simulink model "RudderActuatorChannel_control_lin"  (R2015a)
settings: Solver=ode4  SolverMode=SingleTasking  StartTime=0.0  StopTime=2.999  FixedStep=sampleTime  MaxStep=1e-3  MinStep=1e-4
undefined symbols (not defined in the file or in its folder): Acv, Aleak1, Aleak2, Aleak3, Aleak4, Aleak5, Aleakext, Aleakint, Ap, Ap_seal, Ar_seal, As_ehsv, Be, Bkp_seal, Bp1, C, Cd, ControlTopology, DeltaQ_ehsv, EHSV_Step, ent_air, frictionstribeck_velocity, gamma_air, i_ehsv, Imax, Input, K2_ehsv, K3_ehsv, K_Supply1, Ka1, Kd, Ki, Ki_ehsv, Kp, Kr_ehsv, ksi_ehsv, Kst, Kst_Enable, Kw_ehsv, L0, Load_cmd, Lp_seal, Lr_seal, Max_Cmd, Min_Cmd, Mp1, ON_OFF_hyst, P10, Pcvac, Pcvi, Pcvr, Ps0, Pt0, Ql_ehsv, R, Rate_Limit, Return_Pressure, Rho, sampleTime, seal_compression ... (+20)
undefined symbols (not defined in the file): dpLVDT, Kd_N, ramLVDT, xvLVDT
libraries: simulink x1
(part 1 of 2)
settings Model: SimulationMode=accelerator  Creator=Charles  LastModifiedBy=Pedro H
settings SolverCC: InitialStep=1e-4
settings DataIOCC: LimitDataPoints=off  SaveFormat=StructureWithTime  DSMLogging=off  SaveTime=off
settings OptimizationCC: ExpressionDepthLimit=2147483647  InitFltsAndDblsToZero=on
settings DebuggingCC: SaveWithParameterizedLinksMsg=none  UnderspecifiedInitializationDetection=Classic  MergeDetectMultiDrivingBlocksExec=none  SolverPrmCheckMsg=warning  InheritedTsInSrcMsg=none  FcnCallInpInsideContextMsg=UseLocalSettings  StateNameClashWarn=warning
settings ModelReferenceCC: UpdateModelReferenceTargets=IfOutOfDate
settings GRTTargetCC: TargetFcnLib=ansi_tfl_tmw.mat  CombineOutputUpdateFcns=off  GRTInterface=on

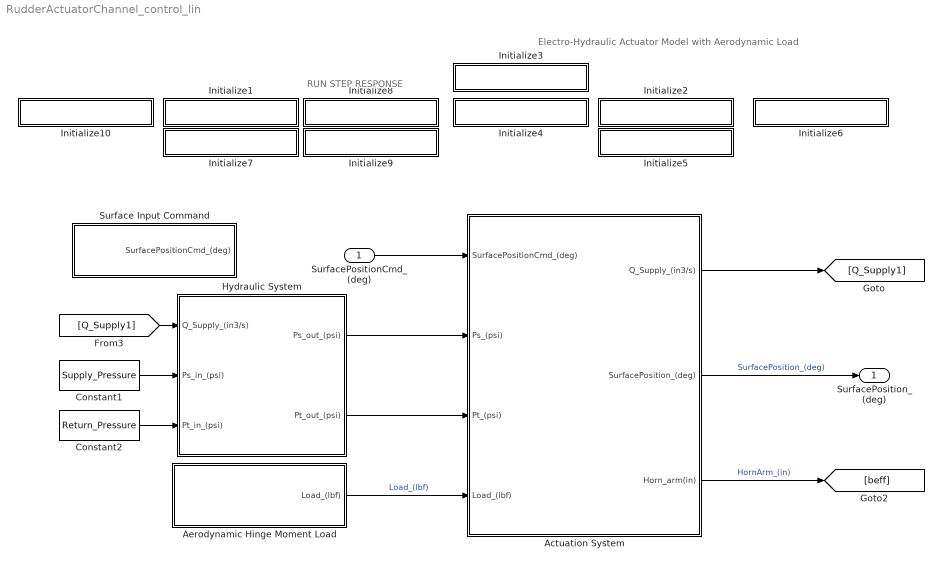
== system RudderActuatorChannel_control_lin ==
  note: RUN STEP RESPONSE
  note: Electro-Hydraulic Actuator Model with Aerodynamic Load
  SurfacePositionCmd_(deg) : Inport
  Actuation System : Subsystem
  Aerodynamic Hinge Moment Load : Subsystem
  Constant1 : Constant  Value=Supply_Pressure
  Constant2 : Constant  Value=Return_Pressure
  Hydraulic System : Subsystem
  Initialize1 : Subsystem
      settings: OpenFcn=|
      | run('StepInput_CLLoad.m'),
      | set_param(bdroot,'SimulationCommand','start')
      mask Display: disp('Closed Loop - Loaded')
  Initialize10 : Subsystem
      settings: OpenFcn=|
      | run('SineInput_CLLoad.m'),
      | set_param(bdroot,'SimulationCommand','start')
      mask Display: disp('Run Sine Input')
  Initialize2 : Subsystem
      settings: OpenFcn=|
      | FreqResp_type = 0;
      | run('FrequencyResponseTest.m'),
      | set_param(bdroot,'SimulationCommand','start')
      mask Display: disp('Frequency Response')
  Initialize3 : Subsystem
      settings: OpenFcn=run('Load_Parameters.m'),
      mask Display: disp('Model Initialization')
  Initialize4 : Subsystem
      settings: OpenFcn=run('plotMaster.m')
      mask Display: disp('Plot Results')
  Initialize5 : Subsystem
      settings: OpenFcn=|
      | FreqResp_type = 1;
      | run('FrequencyResponseTest.m'),
      | set_param(bdroot,'SimulationCommand','start')
      mask Display: disp('Run EHSV Frequency Response Test')
  Initialize6 : Subsystem
      settings: OpenFcn=run('DynamicStiffnessTest.m')
      mask Display: disp('Dynamic Stiffness Test')
  Initialize7 : Subsystem
      settings: OpenFcn=|
      | run('StepInput_CLNoLoad.m'),
      | set_param(bdroot,'SimulationCommand','start')
      mask Display: disp('Closed Loop - Unloaded')
  Initialize8 : Subsystem
      settings: OpenFcn=|
      | run('StepInput_OLEHSVLoad.m'),
      | set_param(bdroot,'SimulationCommand','start')
      mask Display: disp('Open Loop - Loaded')
  Initialize9 : Subsystem
      settings: OpenFcn=|
      | run('StepInput_OLEHSVNoLoad.m'),
      | set_param(bdroot,'SimulationCommand','start')
      mask Display: disp('Open Loop - Unloaded')
  Surface Input Command : Subsystem
  SurfacePosition_(deg) : Outport
  wires:
  Constant1/1 -> Hydraulic System/2(Ps_in_(psi))
  Constant2/1 -> Hydraulic System/3(Pt_in_(psi))
  Hydraulic System/1(Ps_out_(psi)) -> Actuation System/2(Ps_(psi))
  Hydraulic System/2(Pt_out_(psi)) -> Actuation System/3(Pt_(psi))
  Actuation System/1(Q_Supply_(in3/s)) -> [Q_Supply1]
  [Q_Supply1] -> Hydraulic System/1(Q_Supply_(in3/s))
  Actuation System/2(SurfacePosition_(deg)) -> SurfacePosition_(deg)/1  "SurfacePosition_(deg)"
  Actuation System/3(Horn_arm(in)) -> [beff]  "HornArm_(in)"
  Aerodynamic Hinge Moment Load/1(Load_(lbf)) -> Actuation System/4(Load_(lbf))  "Load_(lbf)"
  SurfacePositionCmd_(deg)/1 -> Actuation System/1(SurfacePositionCmd_(deg))

== system RudderActuatorChannel_control_lin/Actuation System ==
  SurfacePositionCmd_(deg) : Inport
  Ps_(psi) : Inport  Port=2
  Pt_(psi) : Inport  Port=3
  Load_(lbf) : Inport  Port=4
  Actuator : Subsystem
  Bus Creator : BusCreator  Inputs=2  OutDataTypeStr=Bus: ActSysHydPower  NonVirtualBus=on
  Electronics System : Subsystem
  Scope : Scope
      settings: SaveName=ScopeData6
  Surface Kinematics : Subsystem
  Q_Supply_(in3/s) : Outport
  SurfacePosition_(deg) : Outport  Port=2
  Horn_arm(in) : Outport  Port=3
  wires:
  [Sensors_FB] -> Electronics System/2(Sensors_FB)
  SurfacePositionCmd_(deg)/1 -> Electronics System/1(Theta_Cmd_(deg))
  Ps_(psi)/1 -> Bus Creator/1  "Ps"
  Pt_(psi)/1 -> Bus Creator/2  "Pt"
  Bus Creator/1 -> Actuator/3(Hyd_Power)
  Actuator/2(Q_Supply) -> Q_Supply_(in3/s)/1
  Actuator/1(Xp_real_(in)) -> Surface Kinematics/1(Xp_(in))  "Xp"
  Load_(lbf)/1 -> [Load]
  Surface Kinematics/1(ThetaPos_(deg)) -> SurfacePosition_(deg)/1
  Actuator/3(Sensors) -> [Sensors_FB]
  Surface Kinematics/2(Effective_arm_(in)) -> Horn_arm(in)/1
  [Load] -> Scope/1, Actuator/2(Load)
  Electronics System/1(Current_Cmd_(mA)) -> Actuator/1(Current_Cmd)

== system RudderActuatorChannel_control_lin/Aerodynamic Hinge Moment Load ==
  Constant2 : Constant  Value=Load_cmd
  Load_(lbf) : Outport
  wires:
  Constant2/1 -> Load_(lbf)/1

== system RudderActuatorChannel_control_lin/Hydraulic System ==
  Q_Supply_(in3/s) : Inport
  Ps_in_(psi) : Inport  Port=2
  Pt_in_(psi) : Inport  Port=3
  Aircraft Hydraulic Losses : Gain  Gain=K_Supply1
  Bus Selector : BusSelector  OutputSignals=Qs
  Fluid Inertia : TransferFcn  Denominator=[0.01 1]
  Sum1 : Sum  Inputs=|+-
  cis to gpm : Gain  Gain=0.25974
  Ps_out_(psi) : Outport
  Pt_out_(psi) : Outport  Port=2
  wires:
  Sum1/1 -> Ps_out_(psi)/1  "Ps"
  Aircraft Hydraulic Losses/1 -> Fluid Inertia/1
  Fluid Inertia/1 -> Sum1/2
  Pt_in_(psi)/1 -> Pt_out_(psi)/1  "Pt"
  Ps_in_(psi)/1 -> Sum1/1  "Ps"
  Q_Supply_(in3/s)/1 -> Bus Selector/1
  cis to gpm/1 -> Aircraft Hydraulic Losses/1
  Bus Selector/1 -> cis to gpm/1  "<Qs>"

== system RudderActuatorChannel_control_lin/Initialize1 ==

== system RudderActuatorChannel_control_lin/Initialize10 ==

== system RudderActuatorChannel_control_lin/Initialize2 ==

== system RudderActuatorChannel_control_lin/Initialize3 ==

== system RudderActuatorChannel_control_lin/Initialize4 ==

== system RudderActuatorChannel_control_lin/Initialize5 ==

== system RudderActuatorChannel_control_lin/Initialize6 ==

== system RudderActuatorChannel_control_lin/Initialize7 ==

== system RudderActuatorChannel_control_lin/Initialize8 ==

== system RudderActuatorChannel_control_lin/Initialize9 ==

== system RudderActuatorChannel_control_lin/Surface Input Command ==
  Step1 : Step  Time=Input.Step.Time  Before=Input.Step.InitialValue  After=Input.Step.FinalValue  SampleTime=0
  SurfacePositionCmd_(deg) : Outport
  wires:
  Step1/1 -> SurfacePositionCmd_(deg)/1

== system RudderActuatorChannel_control_lin/Actuation System/Actuator ==
  Current_Cmd : Inport
  Load : Inport  Port=2
  Hyd_Power : Inport  Port=3
  Cylinder Dynamics : Subsystem
  Sensors Dynamics : Subsystem
  Valves Dynamics : Subsystem
  Xp_real_(in) : Outport
  Q_Supply : Outport  Port=2
  Sensors : Outport  Port=3
  wires:
  Cylinder Dynamics/2(Xp) -> Xp_real_(in)/1, [Xp]
  Load/1 -> Cylinder Dynamics/2(Load)
  Valves Dynamics/2(Q_Supply) -> Q_Supply/1
  Valves Dynamics/1(Q_Act) -> Cylinder Dynamics/1(Q_Act)
  Current_Cmd/1 -> Valves Dynamics/2(Currrent)
  Hyd_Power/1 -> Valves Dynamics/3(Hyd_Pwr)
  Cylinder Dynamics/1(P_Act) -> Valves Dynamics/1(P_Act)
  Cylinder Dynamics/3(Qacv) -> Valves Dynamics/4(Qacv)
  Valves Dynamics/3(Pt) -> Cylinder Dynamics/3(Pt)
  Valves Dynamics/4(Xv_(in)) -> [Xv]
  Cylinder Dynamics/4(dP) -> [dP]
  [Xp] -> Sensors Dynamics/1(Xp)
  [dP] -> Sensors Dynamics/2(dP)
  [Xv] -> Sensors Dynamics/3(Xv)
  Sensors Dynamics/1(Sensors) -> Sensors/1

== system RudderActuatorChannel_control_lin/Actuation System/Electronics System ==
  Theta_Cmd_(deg) : Inport
  Sensors_FB : Inport  Port=2
  Digital Controller : Subsystem
  Hardware_in : Subsystem
  Hardware_out : Subsystem
  Current_Cmd_(mA) : Outport
  wires:
  Theta_Cmd_(deg)/1 -> Hardware_in/1(Theta_Cmd_in)
  Digital Controller/1(EHSV_Cmd) -> Hardware_out/1(EHSV_Cmd_in)
  Hardware_in/1(Theta_Cmd_out) -> Digital Controller/1(Cmd_D)
  Hardware_in/2(Sensors_FB_out) -> Digital Controller/2(Sensors_FB)
  Sensors_FB/1 -> Hardware_in/2(Sensors_FB_in)
  Hardware_out/1(EHSV_Cmd_out) -> Current_Cmd_(mA)/1

== system RudderActuatorChannel_control_lin/Actuation System/Surface Kinematics ==
  Xp_(in) : Inport
  Rad2Deg : Gain  Gain=180/pi  SaturateOnIntegerOverflow=on  OutDataTypeStr=Inherit: Same as input  ParamDataTypeStr=Inherit: Same as input
  Real Kinematics : Subsystem
  ThetaPos_(deg) : Outport
  Effective_arm_(in) : Outport  Port=2
  wires:
  Xp_(in)/1 -> Real Kinematics/1(Xp)
  Real Kinematics/1(Theta) -> Rad2Deg/1
  Rad2Deg/1 -> ThetaPos_(deg)/1
  Real Kinematics/2(Reff) -> Effective_arm_(in)/1

== system RudderActuatorChannel_control_lin/Actuation System/Actuator/Cylinder Dynamics ==
  Q_Act : Inport
  Load : Inport  Port=2
  Pt : Inport  Port=3
  Bus Creator1 : BusCreator  Inputs=2  OutDataTypeStr=Bus: CYLQacv  NonVirtualBus=on
  Bus Creator3 : BusCreator  Inputs=2  OutDataTypeStr=Bus: CYLPAct  NonVirtualBus=on
  Bus Selector : BusSelector  OutputSignals=Q1,Q2
  Fluid Dynamics : Subsystem
  Piston Dynamics : Subsystem
  Scope : Scope  NumInputPorts=5
      settings: YMin=-5~-5~-5~-5~-5  YMax=5~5~5~5~5  SaveName=ScopeData8
  P_Act : Outport
  Xp : Outport  Port=2
  Qacv : Outport  Port=3
  dP : Outport  Port=4
  wires:
  Bus Creator3/1 -> P_Act/1
  Q_Act/1 -> Bus Selector/1
  Bus Selector/2 -> Fluid Dynamics/4(Q2)  "<Q2>"
  Piston Dynamics/1(Xp) -> [Xp], Xp/1
  Piston Dynamics/2(Xpdot) -> [Xpdot]  "Xpdot"
  [Xp] -> Scope/3, Fluid Dynamics/1(xp)
  [Xpdot] -> Scope/4, Fluid Dynamics/2(xpdot)
  Load/1 -> Piston Dynamics/3(FL)
  Bus Selector/1 -> Fluid Dynamics/3(Q1)  "<Q1>"
  Fluid Dynamics/2(P2) -> Scope/2, Piston Dynamics/2(Pr), Bus Creator3/2  "P2"
  Fluid Dynamics/1(P1) -> Scope/1, Piston Dynamics/1(Pe), Bus Creator3/1  "P1"
  Pt/1 -> Fluid Dynamics/5(Pt)
  Fluid Dynamics/3(Qacv1) -> Bus Creator1/1  "Qacv1"
  Fluid Dynamics/4(Qacv2) -> Bus Creator1/2  "Qacv2"
  Bus Creator1/1 -> Qacv/1
  Fluid Dynamics/5(dP) -> Scope/5, dP/1

== system RudderActuatorChannel_control_lin/Actuation System/Actuator/Sensors Dynamics ==
  Xp : Inport
  dP : Inport  Port=2
  Xv : Inport  Port=3
  Bus Creator : BusCreator  Inputs=3  OutDataTypeStr=Bus: SensorDyn  NonVirtualBus=on
  "Xp LVDT " : Subsystem
  "Xv LVDT " : Subsystem
  "dP LVDT " : Subsystem
  Sensors : Outport
  wires:
  dP/1 -> "dP LVDT "/1(dP_real)
  Xp/1 -> "Xp LVDT "/1(Xp_real)
  Xv/1 -> "Xv LVDT "/1(Xv_real)
  "Xv LVDT "/1(Xv_LVDT) -> Bus Creator/3  "Xv_mesured_(in)"
  "dP LVDT "/1(dP_LVDT) -> Bus Creator/2  "dP_mesured_(psi)"
  "Xp LVDT "/1(Xp_LVDT) -> Bus Creator/1  "Xp_mesured_(in)"
  Bus Creator/1 -> Sensors/1

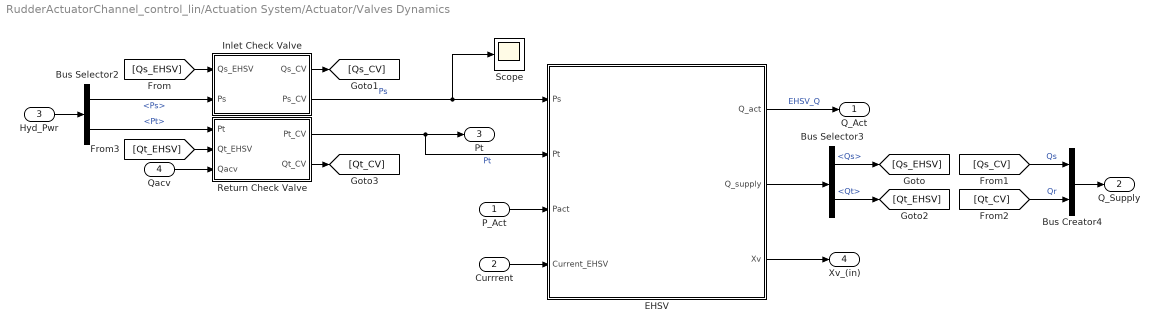
== system RudderActuatorChannel_control_lin/Actuation System/Actuator/Valves Dynamics ==
  P_Act : Inport
  Currrent : Inport  Port=2
  Hyd_Pwr : Inport  Port=3
  Qacv : Inport  Port=4
  Bus Creator4 : BusCreator  Inputs=2  OutDataTypeStr=Bus: VALVEOutQSup  NonVirtualBus=on
  Bus Selector2 : BusSelector  OutputSignals=Ps,Pt
  Bus Selector3 : BusSelector  OutputSignals=Qs,Qt
  EHSV : Subsystem
  Inlet Check Valve : Subsystem
  Return Check Valve : Subsystem
  Scope : Scope
      settings: SaveName=ScopeData5
  Q_Act : Outport
  Q_Supply : Outport  Port=2
  Pt : Outport  Port=3
  Xv_(in) : Outport  Port=4
  wires:
  Hyd_Pwr/1 -> Bus Selector2/1
  EHSV/1(Q_act) -> Q_Act/1  "EHSV_Q"
  Bus Selector2/1 -> Inlet Check Valve/2(Ps)  "<Ps>"
  Bus Selector3/1 -> [Qs_EHSV]  "<Qs>"
  [Qs_EHSV] -> Inlet Check Valve/1(Qs_EHSV)
  Inlet Check Valve/1(Qs_CV) -> [Qs_CV]
  [Qs_CV] -> Bus Creator4/1  "Qs"
  Bus Creator4/1 -> Q_Supply/1
  Bus Selector2/2 -> Return Check Valve/1(Pt)  "<Pt>"
  Bus Selector3/2 -> [Qt_EHSV]  "<Qt>"
  [Qt_CV] -> Bus Creator4/2  "Qr"
  [Qt_EHSV] -> Return Check Valve/2(Qt_EHSV)
  Return Check Valve/2(Qt_CV) -> [Qt_CV]
  Qacv/1 -> Return Check Valve/3(Qacv)
  Currrent/1 -> EHSV/4(Current_EHSV)
  P_Act/1 -> EHSV/3(Pact)
  Inlet Check Valve/2(Ps_CV) -> Scope/1, EHSV/1(Ps)  "Ps"
  Return Check Valve/1(Pt_CV) -> EHSV/2(Pt), Pt/1  "Pt"
  EHSV/2(Q_supply) -> Bus Selector3/1
  EHSV/3(Xv) -> Xv_(in)/1

== system RudderActuatorChannel_control_lin/Actuation System/Electronics System/Digital Controller ==
  Cmd_D : Inport
  Sensors_FB : Inport  Port=2
  Bus Selector : BusSelector  OutputSignals=Xp_FB
  Command Limits : Saturate  UpperLimit=Max_Cmd  LowerLimit=Min_Cmd
  Constant : Constant  Value=ControlTopology
  Constant1 : Constant
  Constant2 : Constant  Value=2
  Deg2Rad : Gain  Gain=pi/180  SampleTime=T_ES  SaturateOnIntegerOverflow=on  OutDataTypeStr=Inherit: Same as input  ParamDataTypeStr=Inherit: Same as input
  Kinematics : Subsystem
  LQR : Subsystem  mask{K=[14.6507 0.0003   22.9112 ]}
      mask prompts: K "State Control gain (K)"
  Manual Switch : ManualSwitch  CurrentSetting=0
  Multiport Switch : MultiPortSwitch  Inputs=5
  On-Off Controller : Relay  OnSwitchValue=ON_OFF_hyst  OffSwitchValue=-ON_OFF_hyst  OnOutputValue=10  OffOutputValue=-10
  PID controller : Subsystem  mask{Kp=Kp, Ki=Ki, Kd=Kd, Ts=T_ES, kd_N=Kd_N, umax=10}
      mask prompts: Ts "Sampling Time"; kd_N "Kd Filter coefficient"; umax "Max command"
  Rate Limit : Subsystem
  Saturation +/- 10mA : Saturate  UpperLimit=Imax  LowerLimit=-Imax  SampleTime=T_ES
  Scope : Scope
  Scope1 : Scope
      settings: SaveName=ScopeData2
  Sgn Convention : Gain  SampleTime=T_ES  SaturateOnIntegerOverflow=on  OutDataTypeStr=Inherit: Same as input  ParamDataTypeStr=Inherit: Same as input
  Step : Step  Time=EHSV_Step.time  Before=EHSV_Step.initial  After=EHSV_Step.final
  Sum : Sum  Inputs=|+-  SampleTime=T_ES  SaturateOnIntegerOverflow=on  InputSameDT=on  OutDataTypeStr=Inherit: Same as first input
  EHSV_Cmd : Outport
  wires:
  Cmd_D/1 -> Rate Limit/1(Cmd)
  Kinematics/1(Xp) -> Sum/1, LQR/1(Ref), Scope1/1  "Pos_Cmd"
  Saturation +/- 10mA/1 -> EHSV_Cmd/1
  Sum/1 -> On-Off Controller/1, PID controller/1(e)  "Pos_Error"
  Command Limits/1 -> Sgn Convention/1
  Deg2Rad/1 -> Kinematics/1(ThetaS)
  Rate Limit/1(Cmd_RL) -> Command Limits/1
  Sgn Convention/1 -> Deg2Rad/1
  Sensors_FB/1 -> Bus Selector/1, LQR/2(y)
  Bus Selector/1 -> Sum/2  "<Xp_FB>"
  Multiport Switch/1 -> Scope/1, Saturation +/- 10mA/1
  Constant/1 -> Manual Switch/2
  On-Off Controller/1 -> Multiport Switch/2
  Constant1/1 -> Multiport Switch/4
  PID controller/1(u) -> Multiport Switch/3
  Step/1 -> Multiport Switch/5
  Manual Switch/1 -> Multiport Switch/1
  Constant2/1 -> Manual Switch/1
  LQR/1(u) -> Multiport Switch/6

== system RudderActuatorChannel_control_lin/Actuation System/Electronics System/Hardware_in ==
  Theta_Cmd_in : Inport
  Sensors_FB_in : Inport  Port=2
  Bus Creator : BusCreator  Inputs=3  OutDataTypeStr=Bus: SensorsFB  NonVirtualBus=on
  Bus Selector : BusSelector  OutputSignals=Xp_FB,dP_FB,Xv_FB
  Rate Transition{2..5} (4 alike) : RateTransition  Deterministic=off  OutPortSampleTime=T_ES
  Signal Processing : Subsystem
  Theta_Cmd_out : Outport
  Sensors_FB_out : Outport  Port=2
  wires:
  Bus Creator/1 -> Sensors_FB_out/1
  Theta_Cmd_in/1 -> Rate Transition2/1
  Rate Transition2/1 -> Theta_Cmd_out/1
  Sensors_FB_in/1 -> Signal Processing/1(Sesnsors_In)
  Bus Selector/1 -> Rate Transition3/1  "<Xp_FB>"
  Rate Transition3/1 -> Bus Creator/1  "Xp_FB"
  Rate Transition4/1 -> Bus Creator/2  "dP_FB"
  Rate Transition5/1 -> Bus Creator/3  "Xv_FB"
  Bus Selector/2 -> Rate Transition4/1  "<dP_FB>"
  Bus Selector/3 -> Rate Transition5/1  "<Xv_FB>"
  Signal Processing/1(Sensors_Out) -> Bus Selector/1

== system RudderActuatorChannel_control_lin/Actuation System/Electronics System/Hardware_out ==
  EHSV_Cmd_in : Inport
  Rate Transition : RateTransition  Deterministic=off  OutPortSampleTime=0
  Servoamplifier Dynamics : TransferFcn  Numerator=[100]  Denominator=[1 100]
  Servoamplifier Tolerance : Gain  Gain=Tol_SA1
  EHSV_Cmd_out : Outport
  wires:
  Rate Transition/1 -> Servoamplifier Dynamics/1
  Servoamplifier Dynamics/1 -> Servoamplifier Tolerance/1
  EHSV_Cmd_in/1 -> Rate Transition/1
  Servoamplifier Tolerance/1 -> EHSV_Cmd_out/1  "Current"

== system RudderActuatorChannel_control_lin/Actuation System/Surface Kinematics/Real Kinematics ==
  Xp : Inport
  Bus Creator : BusCreator  OutDataTypeStr=Bus: RealKin  NonVirtualBus=on
  Bus Selector2 : BusSelector  OutputSignals=C,R,L
  Bus Selector3 : BusSelector  OutputSignals=L,C,R
  Bus Selector4 : BusSelector  OutputSignals=Theta0
  Bus Selector5 : BusSelector  OutputSignals=C
  Constant : Constant  Value=L0
  Constant1 : Constant  Value=R
  Constant2 : Constant  Value=C
  Constant3 : Constant  Value=Theta0
  Law of cosines Get angle : Subsystem
  Law of cosines Get angle1 : Subsystem
  Product : Product  RndMeth=Zero
  Sum1 : Sum  Inputs=++|
  Sum4 : Sum  Inputs=|+-
  Trigonometric Function : Trigonometry
  Theta : Outport
  Reff : Outport  Port=2
  wires:
  Bus Selector2/1 -> Law of cosines Get angle1/1(C1)  "<C>"
  Bus Selector2/2 -> Law of cosines Get angle1/2(C2)  "<R>"
  Law of cosines Get angle1/1("Angle ") -> Sum4/1  "theta"
  Bus Selector4/1 -> Sum4/2  "<Theta0>"
  Sum4/1 -> Theta/1
  Xp/1 -> Sum1/1  "Xp"
  Constant/1 -> Sum1/2  "L0"
  Sum1/1 -> Bus Creator/1  "L"
  Constant2/1 -> Bus Creator/2  "C"
  Constant1/1 -> Bus Creator/3  "R"
  Constant3/1 -> Bus Creator/4  "Theta0"
  Law of cosines Get angle/1("Angle ") -> Trigonometric Function/1  "alfa"
  Bus Selector3/1 -> Law of cosines Get angle/1(C1)  "<L>"
  Bus Selector3/2 -> Law of cosines Get angle/2(C2)  "<C>"
  Bus Selector3/3 -> Law of cosines Get angle/3(H)  "<R>"
  Product/1 -> Reff/1  "Reff"
  Bus Selector5/1 -> Product/1  "<C>"
  Trigonometric Function/1 -> Product/2
  Bus Selector2/3 -> Law of cosines Get angle1/3(H)  "<L>"
  Bus Creator/1 -> Bus Selector3/1, Bus Selector5/1, Bus Selector2/1, Bus Selector4/1

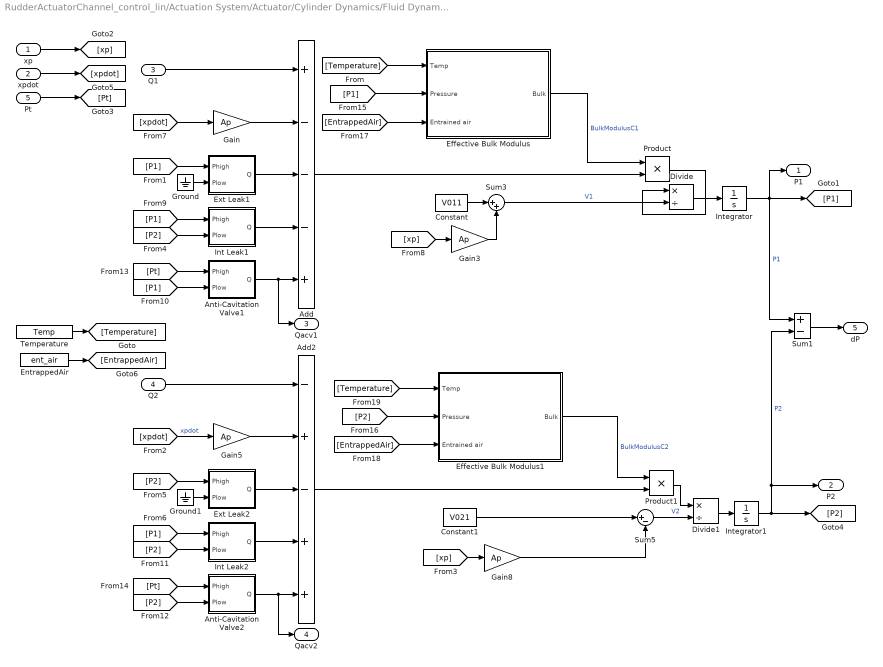
== system RudderActuatorChannel_control_lin/Actuation System/Actuator/Cylinder Dynamics/Fluid Dynamics ==
  xp : Inport
  xpdot : Inport  Port=2
  Q1 : Inport  Port=3
  Q2 : Inport  Port=4
  Pt : Inport  Port=5
  Add : Sum  Inputs=+---+
  Add2 : Sum  Inputs=-+-++
  Anti-Cavitation Valve1 : Subsystem
  Anti-Cavitation Valve2 : Subsystem
  Constant : Constant  Value=V011
  Constant1 : Constant  Value=V021
  Divide : Product  Inputs=*/
  Divide1 : Product  Inputs=*/
  Effective Bulk Modulus : Subsystem
  Effective Bulk Modulus1 : Subsystem
  EntrappedAir : Constant  Value=ent_air
  Ext Leak1 : Subsystem
  Ext Leak2 : Subsystem
  Gain{,3,5,8} (4 alike) : Gain  Gain=Ap
  Ground : Ground
  Ground1 : Ground
  Int Leak1 : Subsystem
  Int Leak2 : Subsystem
  Integrator : Integrator  InitialCondition=P10
  Integrator1 : Integrator  InitialCondition=P10
  Product : Product  RndMeth=Zero
  Product1 : Product  RndMeth=Zero
  Sum1 : Sum  Inputs=+-
  Sum3 : Sum  Inputs=|++
  Sum5 : Sum  Inputs=|+-
  Temperature : Constant  Value=Temp
  P1 : Outport
  P2 : Outport  Port=2
  Qacv1 : Outport  Port=3
  Qacv2 : Outport  Port=4
  dP : Outport  Port=5
  wires:
  Q1/1 -> Add/1
  Q2/1 -> Add2/1
  [xpdot] -> Gain5/1  "xpdot"
  [xp] -> Gain8/1
  Int Leak2/1(Q) -> Add2/4
  Divide1/1 -> Integrator1/1
  Sum5/1 -> Divide1/2  "V2"
  Gain8/1 -> Sum5/2
  Constant1/1 -> Sum5/1
  Integrator1/1 -> [P2], Sum1/2, P2/1  "P2"
  Ext Leak2/1(Q) -> Add2/3
  Gain5/1 -> Add2/2
  Int Leak1/1(Q) -> Add/4
  Divide/1 -> Integrator/1
  Sum3/1 -> Divide/2  "V1"
  Gain3/1 -> Sum3/2
  Constant/1 -> Sum3/1
  Integrator/1 -> Sum1/1, [P1], P1/1  "P1"
  Ext Leak1/1(Q) -> Add/3
  Add/1 -> Product/2
  Gain/1 -> Add/2
  [P1] -> Ext Leak1/1(Phigh)
  [P2] -> Ext Leak2/1(Phigh)
  xpdot/1 -> [xpdot]
  [xpdot] -> Gain/1
  xp/1 -> [xp]
  [xp] -> Gain3/1
  [P2] -> Int Leak1/2(Plow)
  Ground/1 -> Ext Leak1/2(Plow)
  Ground1/1 -> Ext Leak2/2(Plow)
  [P1] -> Int Leak2/1(Phigh)
  [Pt] -> Anti-Cavitation Valve1/1(Phigh)
  [P1] -> Anti-Cavitation Valve1/2(Plow)
  [P1] -> Int Leak1/1(Phigh)
  Anti-Cavitation Valve1/1(Q) -> Add/5, Qacv1/1
  [P2] -> Int Leak2/2(Plow)
  Anti-Cavitation Valve2/1(Q) -> Add2/5, Qacv2/1
  [Pt] -> Anti-Cavitation Valve2/1(Phigh)
  [P2] -> Anti-Cavitation Valve2/2(Plow)
  Pt/1 -> [Pt]
  Product/1 -> Divide/1
  [P1] -> Effective Bulk Modulus/2(Pressure)
  Effective Bulk Modulus/1(Bulk) -> Product/1  "BulkModulusC1"
  Product1/1 -> Divide1/1
  Effective Bulk Modulus1/1(Bulk) -> Product1/1  "BulkModulusC2"
  Add2/1 -> Product1/2
  [P2] -> Effective Bulk Modulus1/2(Pressure)
  Temperature/1 -> [Temperature]
  EntrappedAir/1 -> [EntrappedAir]
  [Temperature] -> Effective Bulk Modulus/1(Temp)
  [EntrappedAir] -> Effective Bulk Modulus/3(Entrained air)
  [EntrappedAir] -> Effective Bulk Modulus1/3(Entrained air)
  [Temperature] -> Effective Bulk Modulus1/1(Temp)
  Sum1/1 -> dP/1

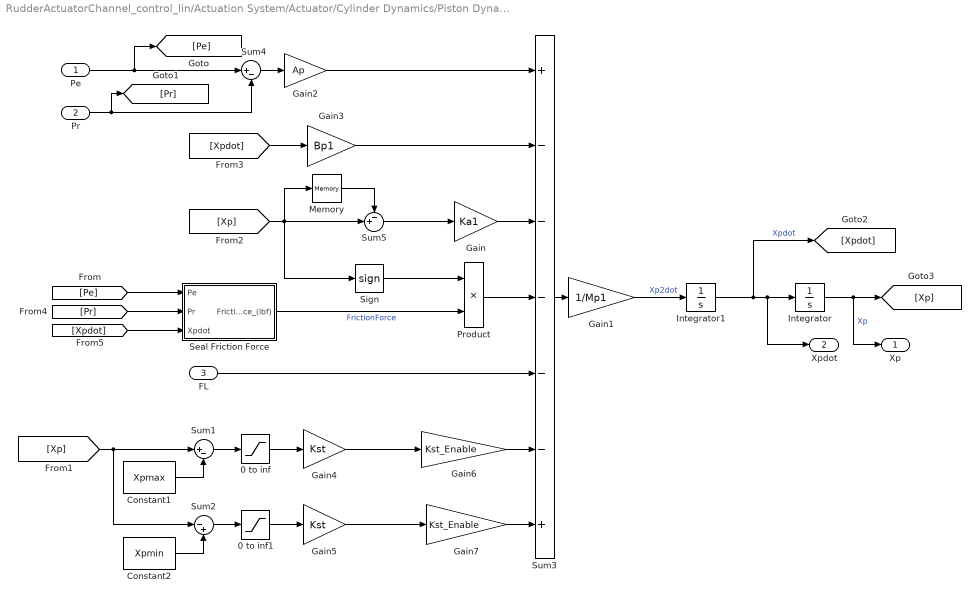
== system RudderActuatorChannel_control_lin/Actuation System/Actuator/Cylinder Dynamics/Piston Dynamics ==
  Pe : Inport
  Pr : Inport  Port=2
  FL : Inport  Port=3
  0 to inf : Saturate  UpperLimit=inf  LowerLimit=0
  0 to inf1 : Saturate  UpperLimit=inf  LowerLimit=0
  Constant1 : Constant  Value=Xpmax
  Constant2 : Constant  Value=Xpmin
  Gain : Gain  Gain=Ka1
  Gain1 : Gain  Gain=1/Mp1
  Gain2 : Gain  Gain=Ap
  Gain3 : Gain  Gain=Bp1
  Gain4 : Gain  Gain=Kst
  Gain5 : Gain  Gain=Kst
  Gain6 : Gain  Gain=Kst_Enable
  Gain7 : Gain  Gain=Kst_Enable
  Integrator : Integrator  InitialCondition=Xp_init
  Integrator1 : Integrator  InitialCondition=0.01
  Memory : Memory
  Product : Product  RndMeth=Zero
  Seal Friction Force : Subsystem
  Sign : Signum
  Sum1 : Sum  Inputs=|+-
  Sum2 : Sum  Inputs=|-+
  Sum3 : Sum  Inputs=+-----+
  Sum4 : Sum  Inputs=|+-
  Sum5 : Sum  Inputs=-+|
  Xp : Outport
  Xpdot : Outport  Port=2
  wires:
  Sum3/1 -> Gain1/1
  Gain1/1 -> Integrator1/1  "Xp2dot"
  Integrator1/1 -> Integrator/1, Xpdot/1, [Xpdot]  "Xpdot"
  Integrator/1 -> [Xp], Xp/1  "Xp"
  [Xp] -> Sign/1, Sum5/2, Memory/1
  Pe/1 -> [Pe], Sum4/1
  Sum4/1 -> Gain2/1
  Gain2/1 -> Sum3/1
  [Xpdot] -> Gain3/1
  Gain3/1 -> Sum3/2
  Gain/1 -> Sum3/3
  FL/1 -> Sum3/5
  Sum1/1 -> 0 to inf/1
  0 to inf/1 -> Gain4/1
  Constant2/1 -> Sum2/2
  Sign/1 -> Product/1
  Product/1 -> Sum3/4
  [Xp] -> Sum1/1, Sum2/1
  Gain4/1 -> Gain6/1
  Sum2/1 -> 0 to inf1/1
  0 to inf1/1 -> Gain5/1
  Gain5/1 -> Gain7/1
  Constant1/1 -> Sum1/2
  Memory/1 -> Sum5/1
  Sum5/1 -> Gain/1
  Seal Friction Force/1(FrictionForce_(lbf)) -> Product/2  "FrictionForce"
  Pr/1 -> [Pr], Sum4/2
  [Pr] -> Seal Friction Force/2(Pr)
  [Pe] -> Seal Friction Force/1(Pe)
  Gain6/1 -> Sum3/6
  Gain7/1 -> Sum3/7
  [Xpdot] -> Seal Friction Force/3(Xpdot)

== system RudderActuatorChannel_control_lin/Actuation System/Actuator/Sensors Dynamics/Xp LVDT  ==
  Xp_real : Inport
  LVDT : Subsystem  mask{band=ramLVDT.Bandwidth, range=ramLVDT.Range, lvdt_error=ramLVDT.Error, hyst=ramLVDT.Hysteresis}
      mask prompts: band "LVDT Bandwdidth"; range "LVDT Range ([min middle max])"; lvdt_error "LVDT error"; hyst "LVDT Hysteresis"
  Xp_LVDT : Outport
  wires:
  Xp_real/1 -> LVDT/1(Sensor In)
  LVDT/1(SensorOut) -> Xp_LVDT/1

== system RudderActuatorChannel_control_lin/Actuation System/Actuator/Sensors Dynamics/Xv LVDT  ==
  Xv_real : Inport
  LVDT1 : Subsystem  mask{band=xvLVDT.Bandwidth, range=xvLVDT.Range, lvdt_error=xvLVDT.Error, hyst=xvLVDT.Hysteresis}
      mask prompts: band "LVDT Bandwdidth (Hz)"; range "LVDT Range ([min middle max])"; lvdt_error "LVDT error"; hyst "LVDT Hysteresis (%)"
  Xv_LVDT : Outport
  wires:
  Xv_real/1 -> LVDT1/1(Sensor In)
  LVDT1/1(SensorOut) -> Xv_LVDT/1

== system RudderActuatorChannel_control_lin/Actuation System/Actuator/Sensors Dynamics/dP LVDT  ==
  dP_real : Inport
  LVDT1 : Subsystem  mask{band=dpLVDT.Bandwidth, range=dpLVDT.Range, lvdt_error=dpLVDT.Error, hyst=dpLVDT.Hysteresis}
      mask prompts: band "LVDT Bandwdidth (Hz)"; range "LVDT Range ([min middle max])"; lvdt_error "LVDT error"; hyst "LVDT Hysteresis (%)"
  dP_LVDT : Outport
  wires:
  dP_real/1 -> LVDT1/1(Sensor In)
  LVDT1/1(SensorOut) -> dP_LVDT/1

== system RudderActuatorChannel_control_lin/Actuation System/Actuator/Valves Dynamics/EHSV ==
  Ps : Inport
  Pt : Inport  Port=2
  Pact : Inport  Port=3
  Current_EHSV : Inport  Port=4
  Bus Selector1 : BusSelector  OutputSignals=P1,P2
  Derivative : Derivative
  EHSV 1st Stage : Subsystem
  EHSV 2nd Stage : Subsystem
  EHSV Test : Subsystem
  EHSV Test1 : Subsystem
  EHSV Test2 : Subsystem
  EHSV Test3 : Subsystem
  EHSV input : Subsystem
  Scope : Scope
  Scope1 : Scope  NumInputPorts=2
      settings: YMin=-5~-5  YMax=5~5  SaveName=ScopeData4
  Q_act : Outport
  Q_supply : Outport  Port=2
  Xv : Outport  Port=3
  wires:
  Bus Selector1/1 -> EHSV Test/1(In1)  "<P1>"
  Bus Selector1/2 -> EHSV Test1/1(In1)  "<P2>"
  EHSV 1st Stage/1(Xv) -> Derivative/1, Xv/1, EHSV 2nd Stage/5(Xv)  "Xv"
  EHSV Test/1(Out1) -> EHSV 2nd Stage/3(P1)  "P1"
  EHSV Test1/1(Out1) -> EHSV 2nd Stage/4(P2)  "P2"
  Pt/1 -> EHSV Test3/1(In1)
  EHSV 2nd Stage/1(Q) -> Q_act/1  "EHSV_Q"
  Ps/1 -> EHSV Test2/1(In1)
  Current_EHSV/1 -> EHSV input/1(CurrentCmd)
  Pact/1 -> Bus Selector1/1
  EHSV 2nd Stage/2(Q_Supply) -> Q_supply/1
  EHSV Test2/1(Out1) -> EHSV 2nd Stage/1(Ps)  "Ps"
  EHSV Test3/1(Out1) -> EHSV 2nd Stage/2(Pt)  "Pt"
  EHSV input/1(EHSV_current) -> EHSV 1st Stage/1(i)  "EHSV_current_cmd"
  EHSV 2nd Stage/3(Q_leak_EHV) -> Scope/1  "Qleak_EHSV"
  Derivative/1 -> Scope1/1, Scope1/2

== system RudderActuatorChannel_control_lin/Actuation System/Actuator/Valves Dynamics/Inlet Check Valve ==
  Qs_EHSV : Inport
  Ps : Inport  Port=2
  Divide : Product  Inputs=*/
  Effective Bulk Modulus : Subsystem
  EntrappedAir : Constant  Value=ent_air
  Inlet Check Valve Flow : Subsystem
  Integrator : Integrator  InitialCondition=Ps0
  Product : Product  RndMeth=Zero
  Sum : Sum  Inputs=-+|
  Temperature : Constant  Value=Temp
  Vcv : Constant  Value=Vcv
  Qs_CV : Outport
  Ps_CV : Outport  Port=2
  wires:
  Inlet Check Valve Flow/1(Q) -> Sum/2, Qs_CV/1
  Qs_EHSV/1 -> Sum/1
  Integrator/1 -> Inlet Check Valve Flow/2(P2), Ps_CV/1
  Sum/1 -> Product/2
  Product/1 -> Integrator/1
  Temperature/1 -> [Temperature]
  EntrappedAir/1 -> [EntrappedAir]
  Ps/1 -> Effective Bulk Modulus/2(Pressure), Inlet Check Valve Flow/1(P1)
  [Temperature] -> Effective Bulk Modulus/1(Temp)
  [EntrappedAir] -> Effective Bulk Modulus/3(Entrained air)
  Divide/1 -> Product/1
  Effective Bulk Modulus/1(Bulk) -> Divide/1
  Vcv/1 -> Divide/2

== system RudderActuatorChannel_control_lin/Actuation System/Actuator/Valves Dynamics/Return Check Valve ==
  Pt : Inport
  Qt_EHSV : Inport  Port=2
  Qacv : Inport  Port=3
  Bus Selector1 : BusSelector  OutputSignals=Qacv1,Qacv2
  Divide : Product  Inputs=*/
  Effective Bulk Modulus : Subsystem
  EntrappedAir : Constant  Value=ent_air
  Integrator : Integrator  InitialCondition=Pt0
  Product : Product  RndMeth=Zero
  Return Check Valve Flow : Subsystem
  Sum : Sum  Inputs=+--
  Sum1 : Sum  Inputs=++|
  Temperature : Constant  Value=Temp
  Vcv : Constant  Value=Vcv
  Pt_CV : Outport
  Qt_CV : Outport  Port=2
  wires:
  Sum/1 -> Product/2
  Integrator/1 -> Return Check Valve Flow/2(P2), Pt_CV/1
  Pt/1 -> Effective Bulk Modulus/2(Pressure), Return Check Valve Flow/1(P1)
  Qt_EHSV/1 -> Sum/1
  Return Check Valve Flow/1(Q) -> Qt_CV/1, Sum/2
  Product/1 -> Integrator/1
  Qacv/1 -> Bus Selector1/1
  Bus Selector1/1 -> Sum1/1  "<Qacv1>"
  Bus Selector1/2 -> Sum1/2  "<Qacv2>"
  Sum1/1 -> Sum/3
  Temperature/1 -> [Temperature]
  EntrappedAir/1 -> [EntrappedAir]
  [Temperature] -> Effective Bulk Modulus/1(Temp)
  [EntrappedAir] -> Effective Bulk Modulus/3(Entrained air)
  Divide/1 -> Product/1
  Effective Bulk Modulus/1(Bulk) -> Divide/1
  Vcv/1 -> Divide/2

== system RudderActuatorChannel_control_lin/Actuation System/Electronics System/Digital Controller/Kinematics ==
  ThetaS : Inport
  Constant : Constant  Value=L0
  Constant1 : Constant  Value=R
  Constant2 : Constant  Value=C
  Constant3 : Constant  Value=Theta0
  Law of cosines Get side : Subsystem
  Sum : Sum  Inputs=|++  SampleTime=T_ES
  Sum1 : Sum  Inputs=|+-  SampleTime=T_ES
  Xp : Outport
  wires:
  ThetaS/1 -> Sum/1  "ThetaS"
  Constant/1 -> Sum1/2  "L0"
  Sum1/1 -> Xp/1
  Constant3/1 -> Sum/2  "Theta0"
  Constant2/1 -> Law of cosines Get side/1(C)  "C"
  Constant1/1 -> Law of cosines Get side/2(R)  "R"
  Sum/1 -> Law of cosines Get side/3(Thetha)
  Law of cosines Get side/1(L) -> Sum1/1

== system RudderActuatorChannel_control_lin/Actuation System/Electronics System/Digital Controller/LQR ==
  Ref : Inport
  y : Inport  Port=2
  Add : Sum  Inputs=|+-
  Add1 : Sum  Inputs=|+-
  Add2 : Sum  Inputs=|++
  Bus Selector : BusSelector  OutputSignals=Xp_FB,dP_FB,Xv_FB
  Gain : Gain  Gain=K(3)
  Gain2 : Gain  Gain=K(1)/K(3)
  Gain3 : Gain  Gain=K(2)/K(3)
  Input control : Scope  NumInputPorts=2
      settings: TimeRange=1.515675675675676  YMin=-5.9091e-26~-400000  YMax=0.0671053~200000  SaveName=ScopeData6
  u : Outport
  wires:
  Ref/1 -> Add/1
  Add/1 -> Input control/1, Add1/1
  Add1/1 -> Input control/2, Gain/1
  Gain/1 -> u/1
  Add2/1 -> Add1/2
  Bus Selector/3 -> Add/2  "<Xv_FB>"
  y/1 -> Bus Selector/1
  Bus Selector/2 -> Gain3/1  "<dP_FB>"
  Bus Selector/1 -> Gain2/1  "<Xp_FB>"
  Gain2/1 -> Add2/1
  Gain3/1 -> Add2/2

== system RudderActuatorChannel_control_lin/Actuation System/Electronics System/Digital Controller/PID controller ==
  e : Inport
  Delay : UnitDelay  SampleTime=-1
  Discrete Transfer Fcn : DiscreteTransferFcn  Numerator=[1 1]  Denominator=[1 -1]
  Discrete Transfer Fcn1 : DiscreteTransferFcn  Numerator=[1 1]  Denominator=[1 -1]
  Filter Coefficient1 : Gain  Gain=Ts/2
  Filter Coefficient2 : Gain  Gain=Ki
  Filter Coefficient3 : Gain  Gain=kd_N
  Filter Coefficient4 : Gain  Gain=Ts/2
  Gain : Gain  Gain=Kp
  Gain1 : Gain  Gain=Ki
  Gain2 : Gain  Gain=Kd
  "Saturation " : Saturate  UpperLimit=umax  LowerLimit=-umax  SampleTime=T_ES
  Sum1 : Sum  Inputs=+++
  Sum2 : Sum  Inputs=-+|
  Sum3 : Sum  Inputs=+-
  Sum4 : Sum  Inputs=|+-
  Unit Delay : UnitDelay  SampleTime=-1
  u : Outport
  wires:
  Gain1/1 -> Sum2/2
  Gain/1 -> Sum1/2
  Sum1/1 -> Sum3/1, "Saturation "/1
  e/1 -> Gain2/1, Gain/1, Gain1/1
  Discrete Transfer Fcn/1 -> Sum1/1
  Filter Coefficient1/1 -> Discrete Transfer Fcn/1
  Gain2/1 -> Sum4/1
  Sum2/1 -> Filter Coefficient1/1
  "Saturation "/1 -> u/1, Sum3/2
  Sum3/1 -> Unit Delay/1
  Filter Coefficient2/1 -> Sum2/1
  Unit Delay/1 -> Filter Coefficient2/1
  Sum4/1 -> Filter Coefficient3/1
  Discrete Transfer Fcn1/1 -> Filter Coefficient4/1
  Filter Coefficient4/1 -> Sum4/2
  Delay/1 -> Discrete Transfer Fcn1/1
  Filter Coefficient3/1 -> Sum1/3, Delay/1

== system RudderActuatorChannel_control_lin/Actuation System/Electronics System/Digital Controller/Rate Limit ==
  Cmd : Inport
  Gain : Gain  Gain=1/T_ES
  Gain1 : Gain  Gain=T_ES
  Rate Limit : Saturate  UpperLimit=Rate_Limit  LowerLimit=-Rate_Limit
  Sum3 : Sum  Inputs=|+-  SaturateOnIntegerOverflow=on  InputSameDT=on  OutDataTypeStr=Inherit: Same as first input
  Sum4 : Sum  Inputs=|++  SaturateOnIntegerOverflow=on  InputSameDT=on  OutDataTypeStr=Inherit: Same as first input
  Unit Delay1 : UnitDelay  SampleTime=-1
  Unit Delay2 : UnitDelay  SampleTime=-1
  Cmd_RL : Outport
  wires:
  Cmd/1 -> Sum3/1
  Unit Delay1/1 -> Sum3/2
  Sum3/1 -> Gain/1  "dCmd"
  Gain/1 -> Rate Limit/1  "Rate"
  Rate Limit/1 -> Gain1/1  "Rate Limited"
  Unit Delay2/1 -> Sum4/2
  Sum4/1 -> Unit Delay2/1, Cmd_RL/1, Unit Delay1/1
  Gain1/1 -> Sum4/1

== system RudderActuatorChannel_control_lin/Actuation System/Electronics System/Hardware_in/Signal Processing ==
  Sesnsors_In : Inport
  Add1 : Sum
  Band-Limited White Noise : simulink/Sources/Band-Limited White Noise  Cov=[0.5]  Ts=sampleTime  seed=[23341]
  Bus Creator : BusCreator  Inputs=3  OutDataTypeStr=Bus: SensorsSP  NonVirtualBus=on
  Bus Selector : BusSelector  OutputSignals=Xp_mesured_(in),dP_mesured_(psi),Xv_mesured_(in)
  RAM LVDT Tolerance : Gain
  Xv LVDT Tolerance : Gain
  dp LVDT Tolerance : Gain
  Sensors_Out : Outport
  wires:
  Sesnsors_In/1 -> Bus Selector/1
  Bus Selector/3 -> Xv LVDT Tolerance/1  "<Xv_mesured_(in)>"
  Bus Selector/1 -> RAM LVDT Tolerance/1  "<Xp_mesured_(in)>"
  Bus Selector/2 -> Add1/1  "<dP_mesured_(psi)>"
  RAM LVDT Tolerance/1 -> Bus Creator/1  "Xp_FB"
  dp LVDT Tolerance/1 -> Bus Creator/2  "dP_FB"
  Xv LVDT Tolerance/1 -> Bus Creator/3  "Xv_FB"
  Bus Creator/1 -> Sensors_Out/1
  Band-Limited White Noise/1 -> Add1/2
  Add1/1 -> dp LVDT Tolerance/1

== system RudderActuatorChannel_control_lin/Actuation System/Surface Kinematics/Real Kinematics/Law of cosines Get angle ==
  C1 : Inport
  C2 : Inport  Port=2
  H : Inport  Port=3
  Add : Sum  Inputs=++-
  Constant4 : Constant  Value=2
  Divide : Product  Inputs=*/
  Math Function : Math  Operator=square  SaturateOnIntegerOverflow=on
  Math Function1 : Math  Operator=square  SaturateOnIntegerOverflow=on
  Math Function2 : Math  Operator=square  SaturateOnIntegerOverflow=on
  Product : Product  Inputs=3
  Trigonometric Function1 : Trigonometry  Operator=acos
  "Angle " : Outport
  wires:
  C1/1 -> Product/2, Math Function/1
  C2/1 -> Product/3, Math Function1/1
  H/1 -> Math Function2/1
  Trigonometric Function1/1 -> "Angle "/1
  Math Function1/1 -> Add/2
  Math Function/1 -> Add/1
  Constant4/1 -> Product/1
  Math Function2/1 -> Add/3
  Add/1 -> Divide/1
  Product/1 -> Divide/2
  Divide/1 -> Trigonometric Function1/1

== system RudderActuatorChannel_control_lin/Actuation System/Surface Kinematics/Real Kinematics/Law of cosines Get angle1 ==
  C1 : Inport
  C2 : Inport  Port=2
  H : Inport  Port=3
  Add : Sum  Inputs=++-
  Constant4 : Constant  Value=2
  Divide : Product  Inputs=*/
  Math Function : Math  Operator=square  SaturateOnIntegerOverflow=on
  Math Function1 : Math  Operator=square  SaturateOnIntegerOverflow=on
  Math Function2 : Math  Operator=square  SaturateOnIntegerOverflow=on
  Product : Product  Inputs=3
  Trigonometric Function1 : Trigonometry  Operator=acos
  "Angle " : Outport
  wires:
  C1/1 -> Product/2, Math Function/1
  C2/1 -> Product/3, Math Function1/1
  H/1 -> Math Function2/1
  Trigonometric Function1/1 -> "Angle "/1
  Math Function1/1 -> Add/2
  Math Function/1 -> Add/1
  Constant4/1 -> Product/1
  Math Function2/1 -> Add/3
  Add/1 -> Divide/1
  Product/1 -> Divide/2
  Divide/1 -> Trigonometric Function1/1

== system RudderActuatorChannel_control_lin/Actuation System/Actuator/Cylinder Dynamics/Fluid Dynamics/Anti-Cavitation Valve1 ==
  Phigh : Inport
  Plow : Inport  Port=2
  Abs : Abs
  Constant : Constant  Value=Acv*sqrt(2/Rho)
  Constant1 : Constant  Value=Pcvac
  Gain : Gain  Gain=Cd/Pcvac
  Math Function : Math  Operator=sqrt  SaturateOnIntegerOverflow=on
  Product : Product  RndMeth=Zero
  Product1 : Product  RndMeth=Zero
  Product2 : Product  RndMeth=Zero
  Saturation : Saturate  UpperLimit=Cd  LowerLimit=0
  Sign : Signum
  Sum : Sum  Inputs=|+-
  Sum1 : Sum  Inputs=|+-
  Q : Outport
  wires:
  Phigh/1 -> Sum/1
  Plow/1 -> Sum/2
  Sum/1 -> Sum1/1, Abs/1, Sign/1
  Constant1/1 -> Sum1/2
  Sum1/1 -> Gain/1
  Gain/1 -> Saturation/1
  Saturation/1 -> Product/1
  Constant/1 -> Product/2
  Abs/1 -> Math Function/1
  Sign/1 -> Product1/1
  Math Function/1 -> Product1/2
  Product1/1 -> Product2/1
  Product/1 -> Product2/2
  Product2/1 -> Q/1

== system RudderActuatorChannel_control_lin/Actuation System/Actuator/Cylinder Dynamics/Fluid Dynamics/Anti-Cavitation Valve2 ==
  Phigh : Inport
  Plow : Inport  Port=2
  Abs : Abs
  Constant : Constant  Value=Acv*sqrt(2/Rho)
  Constant1 : Constant  Value=Pcvac
  Gain : Gain  Gain=Cd/Pcvac
  Math Function : Math  Operator=sqrt  SaturateOnIntegerOverflow=on
  Product : Product  RndMeth=Zero
  Product1 : Product  RndMeth=Zero
  Product2 : Product  RndMeth=Zero
  Saturation : Saturate  UpperLimit=Cd  LowerLimit=0
  Sign : Signum
  Sum : Sum  Inputs=|+-
  Sum1 : Sum  Inputs=|+-
  Q : Outport
  wires:
  Product2/1 -> Q/1
  Product/1 -> Product2/2
  Product1/1 -> Product2/1
  Math Function/1 -> Product1/2
  Sign/1 -> Product1/1
  Abs/1 -> Math Function/1
  Constant/1 -> Product/2
  Saturation/1 -> Product/1
  Gain/1 -> Saturation/1
  Sum1/1 -> Gain/1
  Constant1/1 -> Sum1/2
  Sum/1 -> Sign/1, Abs/1, Sum1/1
  Plow/1 -> Sum/2
  Phigh/1 -> Sum/1

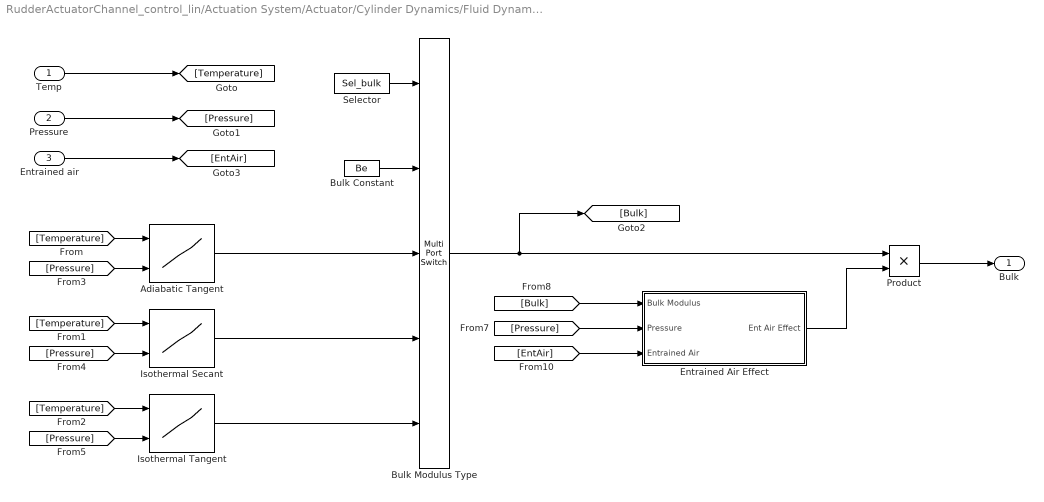
== system RudderActuatorChannel_control_lin/Actuation System/Actuator/Cylinder Dynamics/Fluid Dynamics/Effective Bulk Modulus ==
  Temp : Inport
  Pressure : Inport  Port=2
  Entrained air : Inport  Port=3
  Adiabatic Tangent : Lookup_n-D  BreakpointsForDimension1=[0:10:200]  BreakpointsForDimension2=[1500 3000 5000 8000]  Table=|  RndMeth=Simplest  InputSameDT=on
      | [[328385
      | 317493
      | 306938
      | 296717
      | 286828
      | 277269
      | 268038
      | 259133
      | 250552
      | 242293
      | 234353
      | 226730
      | 219423
      | 212429
      | 205746
      | 199373
      | 193306
      | 187544
      | 182084
      | 176925
      | 172064
      | ],[457660
      | 438564
      | 420172
      | 402478
      | 385479
      | 369170
      | 353546
      | 338602
      | 324335
      | 310740
      | 297812
      | 285547
      | 273940
      | 262986
      | 252681
      | 243021
      | 234001
      | 225616
      | 217863
      | 210735
      | 204230
      | ],[461068
      | 445006
      | 429505
      | 414562
      | 400174
      | 386337
      | 373047
      | 360301
      | 348095
      | 336426
      | 325289
      | 314682
      | 304600
      | 295041
      | 286000
      | 277474
      | 269459
      | 261952
      | 254949
      | 248447
      | 242442
      | ],[531133
      | 516205
      | 501737
      | 487727
      | 474171
      | 461068
      | 448414
      | 436206
      | 424442
      | 413117
      | 402230
      | 391778
      | 381757
      | 372166
      | 363000
      | 354256
      | 345933
      | 338028
      | 330536
      | 323456
      | 316784
      | ]]
  Bulk Constant : Constant  Value=Be
  Bulk Modulus Type : MultiPortSwitch  Inputs=4
  Entrained Air Effect : Subsystem
  Isothermal Secant : Lookup_n-D  BreakpointsForDimension1=[0:10:200]  BreakpointsForDimension2=[0 1500 3000]  Table=|  RndMeth=Simplest  InputSameDT=on
      | [[251501
      | 242817
      | 234410
      | 226279
      | 218424
      | 210846
      | 203544
      | 196518
      | 189768
      | 183295
      | 177098
      | 171177
      | 165533
      | 160165
      | 155073
      | 150257
      | 145718
      | 141455
      | 137468
      | 133757
      | 130323],[259556
      | 251093
      | 242886
      | 234934
      | 227239
      | 219798
      | 212614
      | 205685
      | 199012
      | 192594
      | 186433
      | 180526
      | 174876
      | 169481
      | 164342
      | 159458
      | 154831
      | 150458
      | 146342
      | 142481
      | 138876
      | ],[267611
      | 259369
      | 251362
      | 243590
      | 236053
      | 228751
      | 221684
      | 214852
      | 208255
      | 201894
      | 195767
      | 189875
      | 184219
      | 178797
      | 173611
      | 168660
      | 163943
      | 159462
      | 155216
      | 151205
      | 147429]]
  Isothermal Tangent : Lookup_n-D  BreakpointsForDimension1=[0:10:200]  BreakpointsForDimension2=[0 1500 3000 8000]  Table=|  RndMeth=Simplest  InputSameDT=on
      | [[267611
      | 259369
      | 251362
      | 243590
      | 236053
      | 228751
      | 221684
      | 214852
      | 208255
      | 201894
      | 195767
      | 189875
      | 184219
      | 178797
      | 173611
      | 168660
      | 163943
      | 159462
      | 155216
      | 151205
      | 147429],[372961
      | 358275
      | 344093
      | 330415
      | 317241
      | 304570
      | 292404
      | 280742
      | 269583
      | 258929
      | 248778
      | 239131
      | 229989
      | 221350
      | 213215
      | 205584
      | 198457
      | 191834
      | 185715
      | 180100
      | 174989],[375738
      | 363537
      | 351736
      | 340335
      | 329334
      | 318734
      | 308533
      | 298732
      | 289332
      | 280331
      | 271731
      | 263531
      | 255730
      | 248330
      | 241330
      | 234730
      | 228530
      | 222730
      | 217330
      | 212330
      | 207730],[432836
      | 421701
      | 410889
      | 400400
      | 390232
      | 380388
      | 370866
      | 361667
      | 352790
      | 344236
      | 336004
      | 328095
      | 320508
      | 313244
      | 306303
      | 299684
      | 293388
      | 287414
      | 281763
      | 276434
      | 271428]]
  Product : Product  RndMeth=Zero
  Selector : Constant  Value=Sel_bulk
  Bulk : Outport
  wires:
  Bulk Modulus Type/1 -> [Bulk], Product/1
  Selector/1 -> Bulk Modulus Type/1
  Isothermal Tangent/1 -> Bulk Modulus Type/5
  Isothermal Secant/1 -> Bulk Modulus Type/4
  Bulk Constant/1 -> Bulk Modulus Type/2
  Adiabatic Tangent/1 -> Bulk Modulus Type/3
  Temp/1 -> [Temperature]
  [Temperature] -> Adiabatic Tangent/1
  [Temperature] -> Isothermal Secant/1
  [Temperature] -> Isothermal Tangent/1
  Pressure/1 -> [Pressure]
  [Pressure] -> Adiabatic Tangent/2
  [Pressure] -> Isothermal Secant/2
  [Pressure] -> Isothermal Tangent/2
  [Pressure] -> Entrained Air Effect/2(Pressure)
  Entrained Air Effect/1(Ent Air Effect) -> Product/2
  [Bulk] -> Entrained Air Effect/1(Bulk Modulus)
  Entrained air/1 -> [EntAir]
  [EntAir] -> Entrained Air Effect/3(Entrained Air)
  Product/1 -> Bulk/1

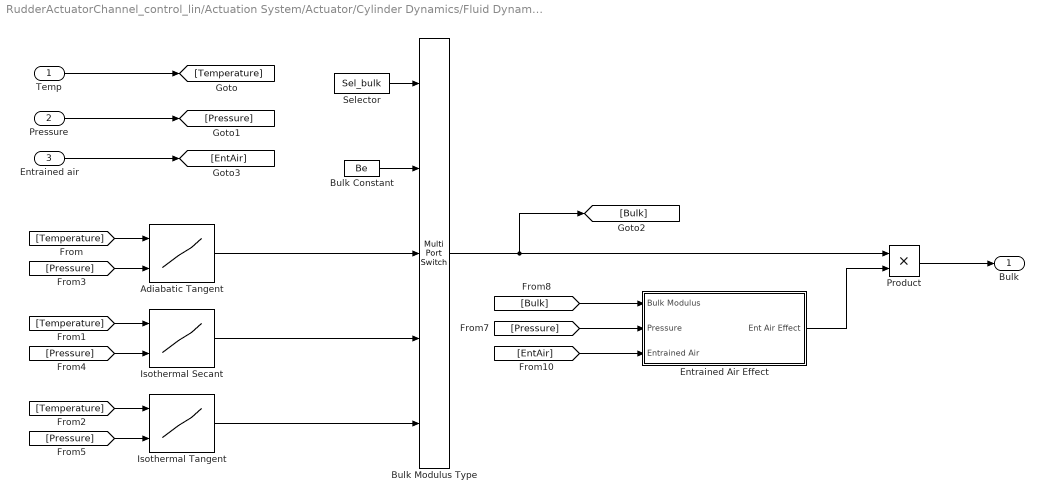
== system RudderActuatorChannel_control_lin/Actuation System/Actuator/Cylinder Dynamics/Fluid Dynamics/Effective Bulk Modulus1 ==
  Temp : Inport
  Pressure : Inport  Port=2
  Entrained air : Inport  Port=3
  Adiabatic Tangent : Lookup_n-D  BreakpointsForDimension1=[0:10:200]  BreakpointsForDimension2=[1500 3000 5000 8000]  Table=|  RndMeth=Simplest  InputSameDT=on
      | [[328385
      | 317493
      | 306938
      | 296717
      | 286828
      | 277269
      | 268038
      | 259133
      | 250552
      | 242293
      | 234353
      | 226730
      | 219423
      | 212429
      | 205746
      | 199373
      | 193306
      | 187544
      | 182084
      | 176925
      | 172064
      | ],[457660
      | 438564
      | 420172
      | 402478
      | 385479
      | 369170
      | 353546
      | 338602
      | 324335
      | 310740
      | 297812
      | 285547
      | 273940
      | 262986
      | 252681
      | 243021
      | 234001
      | 225616
      | 217863
      | 210735
      | 204230
      | ],[461068
      | 445006
      | 429505
      | 414562
      | 400174
      | 386337
      | 373047
      | 360301
      | 348095
      | 336426
      | 325289
      | 314682
      | 304600
      | 295041
      | 286000
      | 277474
      | 269459
      | 261952
      | 254949
      | 248447
      | 242442
      | ],[531133
      | 516205
      | 501737
      | 487727
      | 474171
      | 461068
      | 448414
      | 436206
      | 424442
      | 413117
      | 402230
      | 391778
      | 381757
      | 372166
      | 363000
      | 354256
      | 345933
      | 338028
      | 330536
      | 323456
      | 316784
      | ]]
  Bulk Constant : Constant  Value=Be
  Bulk Modulus Type : MultiPortSwitch  Inputs=4
  Entrained Air Effect : Subsystem
  Isothermal Secant : Lookup_n-D  BreakpointsForDimension1=[0:10:200]  BreakpointsForDimension2=[0 1500 3000]  Table=|  RndMeth=Simplest  InputSameDT=on
      | [[251501
      | 242817
      | 234410
      | 226279
      | 218424
      | 210846
      | 203544
      | 196518
      | 189768
      | 183295
      | 177098
      | 171177
      | 165533
      | 160165
      | 155073
      | 150257
      | 145718
      | 141455
      | 137468
      | 133757
      | 130323],[259556
      | 251093
      | 242886
      | 234934
      | 227239
      | 219798
      | 212614
      | 205685
      | 199012
      | 192594
      | 186433
      | 180526
      | 174876
      | 169481
      | 164342
      | 159458
      | 154831
      | 150458
      | 146342
      | 142481
      | 138876
      | ],[267611
      | 259369
      | 251362
      | 243590
      | 236053
      | 228751
      | 221684
      | 214852
      | 208255
      | 201894
      | 195767
      | 189875
      | 184219
      | 178797
      | 173611
      | 168660
      | 163943
      | 159462
      | 155216
      | 151205
      | 147429]]
  Isothermal Tangent : Lookup_n-D  BreakpointsForDimension1=[0:10:200]  BreakpointsForDimension2=[0 1500 3000 8000]  Table=|  RndMeth=Simplest  InputSameDT=on
      | [[267611
      | 259369
      | 251362
      | 243590
      | 236053
      | 228751
      | 221684
      | 214852
      | 208255
      | 201894
      | 195767
      | 189875
      | 184219
      | 178797
      | 173611
      | 168660
      | 163943
      | 159462
      | 155216
      | 151205
      | 147429],[372961
      | 358275
      | 344093
      | 330415
      | 317241
      | 304570
      | 292404
      | 280742
      | 269583
      | 258929
      | 248778
      | 239131
      | 229989
      | 221350
      | 213215
      | 205584
      | 198457
      | 191834
      | 185715
      | 180100
      | 174989],[375738
      | 363537
      | 351736
      | 340335
      | 329334
      | 318734
      | 308533
      | 298732
      | 289332
      | 280331
      | 271731
      | 263531
      | 255730
      | 248330
      | 241330
      | 234730
      | 228530
      | 222730
      | 217330
      | 212330
      | 207730],[432836
      | 421701
      | 410889
      | 400400
      | 390232
      | 380388
      | 370866
      | 361667
      | 352790
      | 344236
      | 336004
      | 328095
      | 320508
      | 313244
      | 306303
      | 299684
      | 293388
      | 287414
      | 281763
      | 276434
      | 271428]]
  Product : Product  RndMeth=Zero
  Selector : Constant  Value=Sel_bulk
  Bulk : Outport
  wires:
  Bulk Modulus Type/1 -> [Bulk], Product/1
  Selector/1 -> Bulk Modulus Type/1
  Isothermal Tangent/1 -> Bulk Modulus Type/5
  Isothermal Secant/1 -> Bulk Modulus Type/4
  Bulk Constant/1 -> Bulk Modulus Type/2
  Adiabatic Tangent/1 -> Bulk Modulus Type/3
  Temp/1 -> [Temperature]
  [Temperature] -> Adiabatic Tangent/1
  [Temperature] -> Isothermal Secant/1
  [Temperature] -> Isothermal Tangent/1
  Pressure/1 -> [Pressure]
  [Pressure] -> Adiabatic Tangent/2
  [Pressure] -> Isothermal Secant/2
  [Pressure] -> Isothermal Tangent/2
  [Pressure] -> Entrained Air Effect/2(Pressure)
  Entrained Air Effect/1(Ent Air Effect) -> Product/2
  [Bulk] -> Entrained Air Effect/1(Bulk Modulus)
  Entrained air/1 -> [EntAir]
  [EntAir] -> Entrained Air Effect/3(Entrained Air)
  Product/1 -> Bulk/1

== system RudderActuatorChannel_control_lin/Actuation System/Actuator/Cylinder Dynamics/Fluid Dynamics/Ext Leak1 ==
  Phigh : Inport
  Plow : Inport  Port=2
  Abs : Abs
  Constant : Constant  Value=Cd*sqrt(2/Rho)
  Constant3 : Constant  Value=Aleakext
  Math Function : Math  Operator=sqrt  SaturateOnIntegerOverflow=on
  Product : Product  RndMeth=Zero
  Product1 : Product  RndMeth=Zero
  Product3 : Product  RndMeth=Zero
  Sign : Signum
  Sum : Sum  Inputs=|+-
  Q : Outport
  wires:
  Phigh/1 -> Sum/1
  Sum/1 -> Abs/1, Sign/1
  Abs/1 -> Math Function/1
  Sign/1 -> Product/1
  Math Function/1 -> Product/2
  Constant/1 -> Product1/2
  Product/1 -> Product1/1
  Constant3/1 -> Product3/2  "Atot"
  Product1/1 -> Product3/1
  Product3/1 -> Q/1
  Plow/1 -> Sum/2

== system RudderActuatorChannel_control_lin/Actuation System/Actuator/Cylinder Dynamics/Fluid Dynamics/Ext Leak2 ==
  Phigh : Inport
  Plow : Inport  Port=2
  Abs : Abs
  Constant : Constant  Value=Cd*sqrt(2/Rho)
  Constant3 : Constant  Value=Aleakext
  Math Function : Math  Operator=sqrt  SaturateOnIntegerOverflow=on
  Product : Product  RndMeth=Zero
  Product1 : Product  RndMeth=Zero
  Product3 : Product  RndMeth=Zero
  Sign : Signum
  Sum : Sum  Inputs=|+-
  Q : Outport
  wires:
  Plow/1 -> Sum/2
  Product3/1 -> Q/1
  Product1/1 -> Product3/1
  Constant3/1 -> Product3/2  "Atot"
  Product/1 -> Product1/1
  Constant/1 -> Product1/2
  Math Function/1 -> Product/2
  Sign/1 -> Product/1
  Abs/1 -> Math Function/1
  Sum/1 -> Sign/1, Abs/1
  Phigh/1 -> Sum/1

== system RudderActuatorChannel_control_lin/Actuation System/Actuator/Cylinder Dynamics/Fluid Dynamics/Int Leak1 ==
  Phigh : Inport
  Plow : Inport  Port=2
  Abs : Abs
  Constant : Constant  Value=Cd*sqrt(2/Rho)
  Constant3 : Constant  Value=Aleakint
  Math Function : Math  Operator=sqrt  SaturateOnIntegerOverflow=on
  Product : Product  RndMeth=Zero
  Product1 : Product  RndMeth=Zero
  Product3 : Product  RndMeth=Zero
  Sign : Signum
  Sum : Sum  Inputs=|+-
  Q : Outport
  wires:
  Plow/1 -> Sum/2
  Product3/1 -> Q/1
  Product1/1 -> Product3/1
  Constant3/1 -> Product3/2  "Atot"
  Product/1 -> Product1/1
  Constant/1 -> Product1/2
  Math Function/1 -> Product/2
  Sign/1 -> Product/1
  Abs/1 -> Math Function/1
  Sum/1 -> Sign/1, Abs/1
  Phigh/1 -> Sum/1
